simulink model "matmul_comlex"  (R2024a)
settings: Solver=FixedStepDiscrete  StartTime=0.0  StopTime=0.000001  FixedStep=1e-8  RelTol=1e-3
settings Model: Creator=twopi  LastModifiedBy=twopi

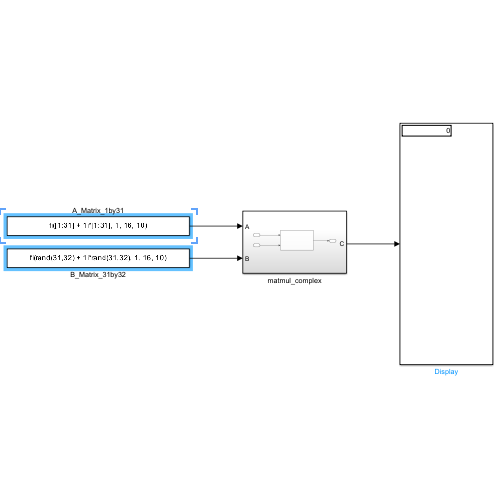
[thumbnail: Simulink's stored preview of the top-level diagram]
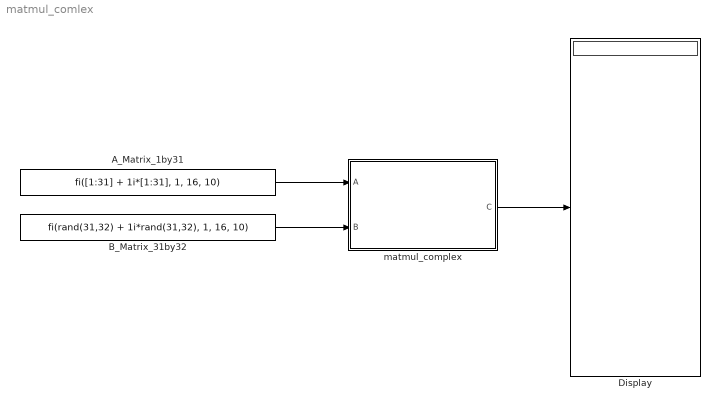
== system matmul_comlex ==
  A_Matrix_1by31 : Constant  Value=fi([1:31] + 1i*[1:31], 1, 16, 10)  VectorParams1D=off  OutDataTypeStr=Inherit: Inherit via back propagation
  B_Matrix_31by32 : Constant  Value=fi(rand(31,32) + 1i*rand(31,32), 1, 16, 10)  OutDataTypeStr=Inherit: Inherit via back propagation
  Display : Display
  matmul_complex : Subsystem
  wires:
  A_Matrix_1by31/1 -> matmul_complex/1(A)
  B_Matrix_31by32/1 -> matmul_complex/2(B)
  matmul_complex/1(C) -> Display/1

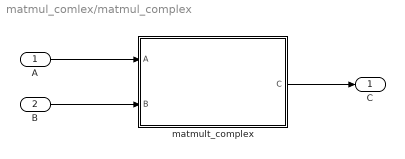
== system matmul_comlex/matmul_complex ==
  A : Inport  OutDataTypeStr=fixdt(1,16,10)
  B : Inport  Port=2  OutDataTypeStr=fixdt(1,16,10)
  matmult_complex : MATLAB Function  TreatAsAtomicUnit=on
  C : Outport
  wires:
  A/1 -> matmult_complex/1(A)
  matmult_complex/1(C) -> C/1
  B/1 -> matmult_complex/2(B)

== matlab function matmul_comlex/matmul_complex/matmult_complex ==
  data: A input; C output; B input
function C = matmul_complex(A, B)
%#codegen
% HDL-friendly matrix multiplication
% A: 1x31, B: 31x32 -> C: 1x32
% Complex fixed-point (sfix16_En10)

% Define types
T_elem = numerictype(1,16,10);   % signed, 16-bit, 10 frac
T_acc  = numerictype(1,32,20);   % accumulator wider
F = fimath('RoundingMethod','Nearest','OverflowAction','Saturate', ...
           'ProductMode','SpecifyPrecision','ProductWordLength',32,'ProductFractionLength',20, ...
           'SumMode','SpecifyPrecision','SumWordLength',32,'SumFractionLength',20);

% Preallocate output as fi (not zeros!)
C = fi(complex(zeros(1,32,'like',fi(0, T_elem, F))), T_elem, F);

% Loop streaming for min resources
coder.hdl.loopspec('stream');

for j = 1:32
    acc = fi(0, T_acc, F) + 1i*fi(0, T_acc, F);  % proper complex fi zero
    for k = 1:31
        prod = A(k) * B(k,j);
        acc  = acc + prod;
    end
    % Cast back to element type
    C(j) = fi(acc, T_elem, F);
end
